simulink model "saturate_int_test"  (Simulink 7.2)
settings: Solver=VariableStepDiscrete  StartTime=0.0  StopTime=10.0  RelTol=1e-3
settings Model: Creator=arnaud  LastModifiedBy=arnaud
settings DataIOCC: SaveFormat=Structure

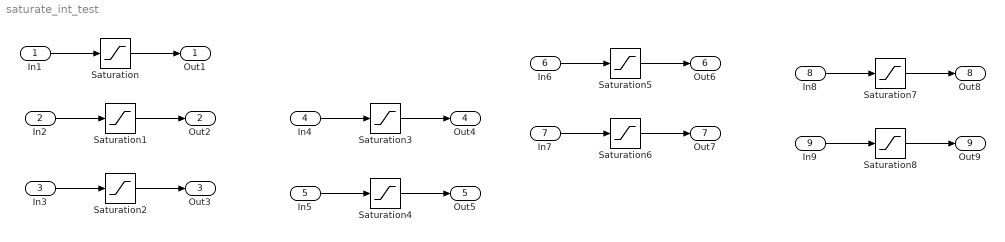
== system saturate_int_test ==
  In1 : Inport  DataType=int8  OutDataType=sfix(16)  OutScaling=2^0  OutDataTypeStr=int8
  In2 : Inport  Port=2  PortDimensions=3  DataType=int8  OutDataType=sfix(16)  OutScaling=2^0  OutDataTypeStr=int8
  In3 : Inport  Port=3  PortDimensions=[2 3]  DataType=int8  OutDataType=sfix(16)  OutScaling=2^0  OutDataTypeStr=int8
  In4 : Inport  Port=4  PortDimensions=3  DataType=int8  OutDataType=sfix(16)  OutScaling=2^0  OutDataTypeStr=int8
  In5 : Inport  Port=5  PortDimensions=[2 3]  DataType=int8  OutDataType=sfix(16)  OutScaling=2^0  OutDataTypeStr=int8
  In6 : Inport  Port=6  DataType=int8  OutDataType=sfix(16)  OutScaling=2^0  OutDataTypeStr=int8
  In7 : Inport  Port=7  DataType=int8  OutDataType=sfix(16)  OutScaling=2^0  OutDataTypeStr=int8
  In8 : Inport  Port=8  DataType=int8  OutDataType=sfix(16)  OutScaling=2^0  OutDataTypeStr=int8
  In9 : Inport  Port=9  DataType=int8  OutDataType=sfix(16)  OutScaling=2^0  OutDataTypeStr=int8
  Saturation : Saturate  UpperLimit=0.6  OutDataType=sfix(16)  OutScaling=2^0
  Saturation1 : Saturate  UpperLimit=0.4  OutDataType=sfix(16)  OutScaling=2^0  RndMeth=Ceiling
  Saturation2 : Saturate  UpperLimit=0.6  OutDataType=sfix(16)  OutScaling=2^0  RndMeth=Nearest
  Saturation3 : Saturate  UpperLimit=[0.4 0.6 0.7]  LowerLimit=[-0.5 -0.6 -0.7]  OutDataType=sfix(16)  OutScaling=2^0  RndMeth=Zero
  Saturation4 : Saturate  UpperLimit=[0.5 0.6 0.7; 1.5 1.6 1.7]  LowerLimit=[-0.5 -0.6 -0.7; -1.5 -1.6 -1.7]  OutDataType=sfix(16)  OutScaling=2^0  RndMeth=Zero
  Saturation5 : Saturate  UpperLimit=[2 3 4]  LowerLimit=[-2 -3 -4]  OutDataType=sfix(16)  OutScaling=2^0
  Saturation6 : Saturate  UpperLimit=[2 3 4; 5 6 7]  LowerLimit=[-2 -3 -4; -5 -6 -7]  OutDataType=sfix(16)  OutScaling=2^0
  Saturation7 : Saturate  UpperLimit=2  LowerLimit=[-2 -3 -4]  OutDataType=sfix(16)  OutScaling=2^0
  Saturation8 : Saturate  UpperLimit=[2 3 4; 5 6 7]  LowerLimit=-2  OutDataType=sfix(16)  OutScaling=2^0
  Out1 : Outport  OutDataType=sfix(16)  OutScaling=2^0
  Out2 : Outport  Port=2  OutDataType=sfix(16)  OutScaling=2^0
  Out3 : Outport  Port=3  OutDataType=sfix(16)  OutScaling=2^0
  Out4 : Outport  Port=4  OutDataType=sfix(16)  OutScaling=2^0
  Out5 : Outport  Port=5  OutDataType=sfix(16)  OutScaling=2^0
  Out6 : Outport  Port=6  OutDataType=sfix(16)  OutScaling=2^0
  Out7 : Outport  Port=7  OutDataType=sfix(16)  OutScaling=2^0
  Out8 : Outport  Port=8  OutDataType=sfix(16)  OutScaling=2^0
  Out9 : Outport  Port=9  OutDataType=sfix(16)  OutScaling=2^0
  wires:
  In1/1 -> Saturation/1
  Saturation/1 -> Out1/1
  In2/1 -> Saturation1/1
  Saturation1/1 -> Out2/1
  In3/1 -> Saturation2/1
  Saturation2/1 -> Out3/1
  In4/1 -> Saturation3/1
  Saturation3/1 -> Out4/1
  In5/1 -> Saturation4/1
  Saturation4/1 -> Out5/1
  In6/1 -> Saturation5/1
  Saturation5/1 -> Out6/1
  In7/1 -> Saturation6/1
  Saturation6/1 -> Out7/1
  In8/1 -> Saturation7/1
  Saturation7/1 -> Out8/1
  In9/1 -> Saturation8/1
  Saturation8/1 -> Out9/1
